simulink model "SADC1"  (R2016b)
settings: Solver=ode4  StartTime=0.0  StopTime=dt_sim  FixedStep=dt_sim  RelTol=1e-3
values from neighbouring files (symbols this model uses):
  I_sc = diag([10000 30000 30000])    [main.m]
  q_bi0 = [0;0;0;1]    [main.m]
  T_ext = [0;0;0]    [main.m]
  w_bi0 = [1;1;0]*d2r    [main.m]
settings Model: Creator=Rich  LastModifiedBy=Rich

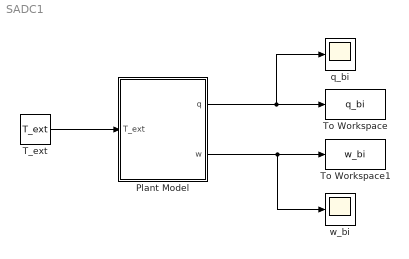
== system SADC1 ==
  Plant Model : Subsystem
  T_ext : Constant  Value=T_ext
  To Workspace : ToWorkspace  VariableName=q_bi  SaveFormat=Timeseries  SampleTime=-1
  To Workspace1 : ToWorkspace  VariableName=w_bi  SaveFormat=Timeseries  SampleTime=-1
  q_bi : Scope
  w_bi : Scope
  wires:
  T_ext/1 -> Plant Model/1(T_ext)
  Plant Model/2(w) -> w_bi/1, To Workspace1/1
  Plant Model/1(q) -> q_bi/1, To Workspace/1

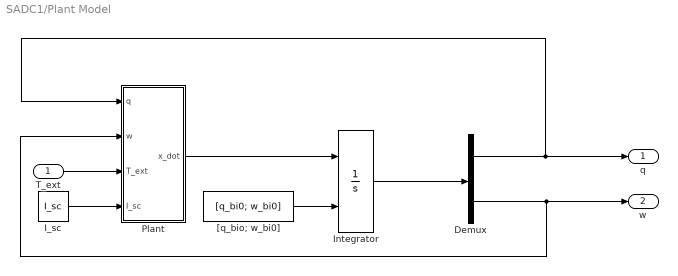
== system SADC1/Plant Model ==
  T_ext : Inport
  Demux : Demux  Outputs=[4 3]
  I_sc : Constant  Value=I_sc
  Integrator : Integrator  InitialConditionSource=external
  Plant : MATLAB Function  TreatAsAtomicUnit=on
  "[q_bio; w_bi0]" : Constant  Value=[q_bi0; w_bi0]
  q : Outport
  w : Outport  Port=2
  wires:
  I_sc/1 -> Plant/4(I_sc)
  Plant/1(x_dot) -> Integrator/1
  "[q_bio; w_bi0]"/1 -> Integrator/2
  Integrator/1 -> Demux/1
  T_ext/1 -> Plant/3(T_ext)
  Demux/2 -> w/1, Plant/2(w)
  Demux/1 -> q/1, Plant/1(q)

== matlab function SADC1/Plant Model/Plant ==
  data: q input; x_dot output; w input; T_ext input; I_sc input
function x_dot = fcn(q,w,T_ext,I_sc)

OMEGA = [0 w(3) -w(2) w(1); -w(3) 0 w(1) w(2); w(2) -w(1) 0 w(3); -w(1) -w(2) -w(3) 0];

q_dot = 0.5*OMEGA*q;

w_dot = inv(I_sc)*(T_ext - cross(w,I_sc*w));

x_dot = [q_dot; w_dot];
